simulink model "Linearni_system_s_regulatorem"  (R2020a)
settings: Solver=VariableStepAuto  StartTime=0.0  StopTime=50  RelTol=1e-3
values from neighbouring files (symbols this model uses):
  dphi = 0    [Model_kyvadla_na_voziku_m.m]
  dx = 0    [Model_kyvadla_na_voziku_m.m]
  f = 10    [Model_kyvadla_na_voziku_m.m]
  K = acker(sys.A, sys.B, [p1, p2, p3, p4])    [Model_kyvadla_na_voziku_m.m]
  phi = deg2rad(1)    [Model_kyvadla_na_voziku_m.m]
  sys = ss(A, B, C, D)    [Model_kyvadla_na_voziku_m.m]
  x = 0    [Model_kyvadla_na_voziku_m.m]
settings Model: Creator=Jiří  LastModifiedBy=Jiří

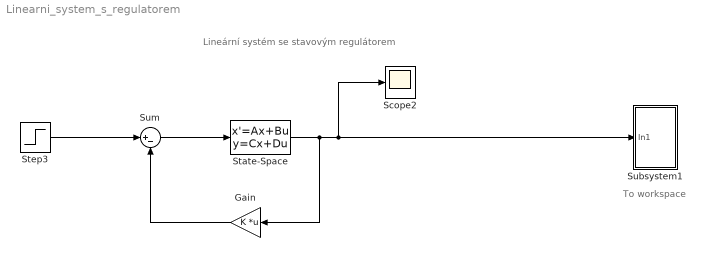
== system Linearni_system_s_regulatorem ==
  note: Lineární systém se stavovým regulátorem
  note: To workspace
  Gain : Gain  Gain=K  Multiplication=Matrix(K*u)
  Scope2 : Scope
  State-Space : StateSpace  A=sys.A  B=sys.B  C=sys.C  D=sys.D  InitialCondition=[x, phi, dx, dphi]
  Step3 : Step  Time=10  After=f  SampleTime=1
  Subsystem1 : Subsystem
  Sum : Sum  Inputs=|+-
  wires:
  Sum/1 -> State-Space/1
  Step3/1 -> Sum/1
  State-Space/1 -> Gain/1, Subsystem1/1(In1), Scope2/1
  Gain/1 -> Sum/2

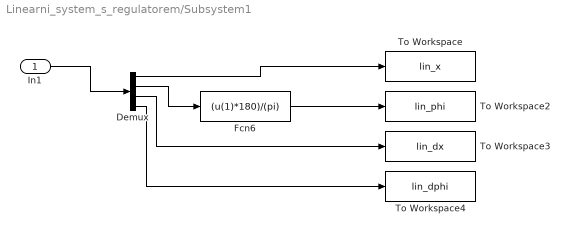
== system Linearni_system_s_regulatorem/Subsystem1 ==
  In1 : Inport
  Demux : Demux
  Fcn6 : Fcn  Expr=(u(1)*180)/(pi)
  To Workspace : ToWorkspace  VariableName=lin_x  SaveFormat=Timeseries  SampleTime=-1
  To Workspace2 : ToWorkspace  VariableName=lin_phi  SaveFormat=Timeseries  SampleTime=-1
  To Workspace3 : ToWorkspace  VariableName=lin_dx  SaveFormat=Timeseries  SampleTime=-1
  To Workspace4 : ToWorkspace  VariableName=lin_dphi  SaveFormat=Timeseries  SampleTime=-1
  wires:
  In1/1 -> Demux/1
  Demux/4 -> To Workspace4/1
  Demux/1 -> To Workspace/1
  Fcn6/1 -> To Workspace2/1
  Demux/2 -> Fcn6/1
  Demux/3 -> To Workspace3/1
